simulink subsystem "TransferCaseSSC"  (R2025b)
settings: Solver=VariableStepAuto  StartTime=0.0  StopTime=10.0  RelTol=1e-3
undefined symbols (not defined in the file): PlntTrnsfrCaseCarrDamp, PlntTrnsfrCaseCompStiff, PlntTrnsfrCaseTrqSplitTimeCnst
libraries: sdl_lib x3, nesl_utility_internal x3, fl_lib x2
settings Model: Creator=The MathWorks, Inc.  LastModifiedBy=The MathWorks, Inc.
settings OptimizationCC: ReuseModelBlockBuffer=off
settings RTWCC: GPUComputeCapability=3.5

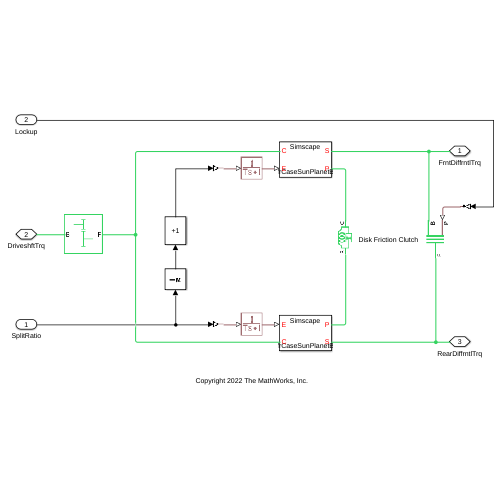
[thumbnail: Simulink's stored preview of the top-level diagram]
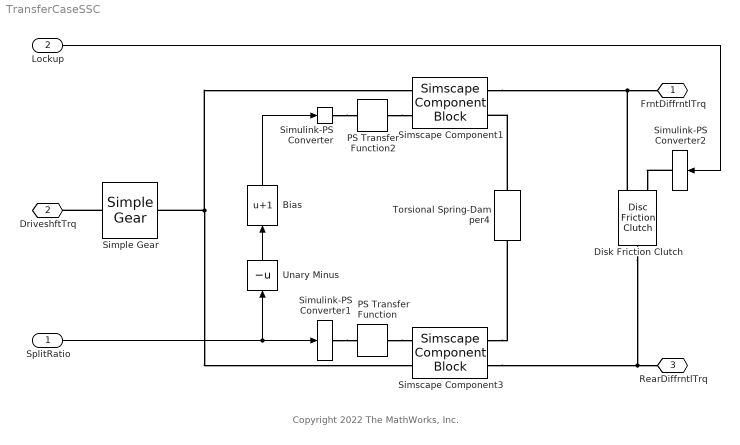
== system TransferCaseSSC ==
  note: Copyright 2022 The MathWorks, Inc.
  SplitRatio : Inport
  Lockup : Inport  Port=2
  Bias : Bias  Bias=1  SaturateOnIntegerOverflow=off
  Disk Friction Clutch : sdl_lib/Clutches/Disc Friction Clutch  geometry_model=sdl.enum.friction_geometry.radius  r_eff=PlntTrnsfrCaseCltchEffRad mm  d_o=150 mm  d_i=100 mm  nS=PlntTrnsfrCaseCltchNumFricSurf  piston_area=PlntTrnsfrCaseCltchEngdPstnArea m^2  unidirectional=sdl.enum.directionality.bidirectional  friction_model=sdl.enum.friction_model_TLU_thermal.fixed  mu_w_vector=[0, 100, 1000] rad/s  temperature_TLU=[280, 300, 320] K  mu_static=PlntTrnsfrCaseCltchStatFric  mu_static_vector=[.4, .38, .36]  mu_coulomb=PlntTrnsfrCaseCltchKinFric  mu_coulomb_vector=[.3, .22, .19]  mu_coulomb_temp_vector=[.3, .28, .25]  mu_coulomb_matrix=[.34, .32, .3; .3, .28, .25; .25, .2, .15]  mu_interp_method=simscape.enum.interpolation.linear  mu_extrap_method=simscape.enum.extrapolation.linear  d_f=PlntTrnsfrCaseCltchDerateFctr  w_tol=PlntTrnsfrCaseCltchVelTol rad/s  pressure_min=PlntTrnsfrCaseCltchEngdThreshPrs Pa  mu_visc=PlntTrnsfrCaseCltchViscDragTrq N*m*s/rad  initial_state_locked=sdl.enum.initial_lock.unlocked  thermal_mass=50 kJ/K  T_init=300 K
      settings: InternalSimscapePortConfiguration="{\"Bottom\":[],\"Left\":[{\"id\":\"P\",\"label\":\"P\",\"type\":\"input\"},{\"id\":\"B\",\"label\":\"B\",\"type\":\"foundation.mechanical.rotational.rotational\"}],\"Right\":[{\"id\":\"F\",\"label\":\"F\",\"type\":\"foundation.mechanical.rotational.rotational\"}],\"Top\":[]}"
  PS Transfer Function : fl_lib/Physical Signals/Linear Operators/PS Transfer Function  transfer_function_type=foundation.enum.transfer_function_type.lag  T=PlntTrnsfrCaseTrqSplitTimeCnst s  T1=2 s  T2=1 s  reset_method=foundation.enum.IntegratorResetSpec.None  initial_condition_spec=foundation.enum.IntegratorICSpec.Internal  y0=PlntTrnsfrCaseTrqSplitRatio
      settings: InternalSimscapePortConfiguration="{\"Bottom\":[],\"Left\":[{\"id\":\"U\",\"label\":\"\",\"type\":\"input\"}],\"Right\":[{\"id\":\"Y\",\"label\":\"\",\"type\":\"output\"}],\"Top\":[]}"
  PS Transfer Function2 : fl_lib/Physical Signals/Linear Operators/PS Transfer Function  transfer_function_type=foundation.enum.transfer_function_type.lag  T=PlntTrnsfrCaseTrqSplitTimeCnst s  T1=2 s  T2=1 s  reset_method=foundation.enum.IntegratorResetSpec.None  initial_condition_spec=foundation.enum.IntegratorICSpec.Internal  y0=PlntTrnsfrCaseTrqSplitRatio
      settings: InternalSimscapePortConfiguration="{\"Bottom\":[],\"Left\":[{\"id\":\"U\",\"label\":\"\",\"type\":\"input\"}],\"Right\":[{\"id\":\"Y\",\"label\":\"\",\"type\":\"output\"}],\"Top\":[]}"
  Simple Gear : sdl_lib/Gears/Simple Gear  ratio=PlntTrnsfrCaseRatio  rotation_direction=sdl.enum.shaftOutputDirection.same  friction_model=sdl.enum.gear_efficiencies_load.constant  T_noload=0.1 N*m  T_nom=5 N*m  efficiency_nom=0.8  efficiency=PlntTrnsfrCaseEff  temperature_TLU=[280, 300, 320] K  load_TLU=[1, 5, 10] N*m  efficiency_TLU=[.95, .9, .85]  efficiency_TLU2=[.85, .8, .75; .95, .9, .85; .85, .8, .7]  w_thr=0.01 rad/s  pwr_thr=PlntTrnsfrCasePwrThresh W  enable_backlash=false  hardstop_model=simscape.enum.hardstop.smooth  backlash_distance=1e-3 mm  r_base=0.1 m  transition=1e-4 mm  backlash_stiffness=1e7 N/m  backlash_damping=1e6 N/(m/s)  coeff_rest=0  v_tol=0.001 m/s  f_tol=0 N  mu_visc=[PlntTrnsfrCaseCarrDamp, PlntTrnsfrCaseCarrDamp] N*m/(rad/s)  thermal_mass=50 J/K  temperature_specify=off  temperature_priority=High  temperature=300 K  temperature_nominal_specify=off  temperature_nominal_value=1  temperature_nominal_unit=K  x_backlash_specify=off  x_backlash_priority=None  x_backlash=0 mm  x_backlash_nominal_specify=off  x_backlash_nominal_value=1  x_backlash_nominal_unit=mm  f_hardstop_specify=off  f_hardstop_priority=None  f_hardstop=0 N  f_hardstop_nominal_specify=off  f_hardstop_nominal_value=1  f_hardstop_nominal_unit=N  v_backlash_specify=off  v_backlash_priority=None  v_backlash=0 m/s  v_backlash_nominal_specify=off  v_backlash_nominal_value=1  v_backlash_nominal_unit=m/s
  Simscape Component1 : SimscapeComponentBlock  SourceFile=TrnsfrCaseSunPlanetBevel  ComponentPath=TrnsfrCaseSunPlanetBevel  ComponentVariants="[\"TrnsfrCaseSunPlanetBevel\"]"  ComponentVariantNames="[\"TrnsfrCaseSunPlanetBevel\"]"  ClassName=TrnsfrCaseSunPlanetBevel  SchemaVersion=1  ratio=PlntTrnsfrCasePlanetSunRatio  assembly_orientation=sdl.enum.sun_planet_bevel_orientation.right  friction_model=sdl.enum.gear_friction.none  efficiency=0.9  temperature_TLU=[280, 300, 320] K  efficiency_TLU=[.95, .9, .85]  pwr_thr=0.001 W  mu_visc=PlntTrnsfrCaseAxl1Damp N*m*s/rad  thermal_mass=50 J/K  temperature_specify=off  temperature_priority=High  temperature=300 K  temperature_nominal_specify=off  temperature_nominal_value=1  temperature_nominal_unit=K
      settings: CopyFcn=simscape.sscblock.internal.componentBlockCallback(gcbh,'COPY')  PreCopyFcn=simscape.sscblock.internal.componentBlockCallback(gcbh,'PRECOPY')  PreDeleteFcn=simscape.sscblock.internal.componentBlockCallback(gcbh,'PREDELETE')  InternalSimscapePortConfiguration="{\"Bottom\":[],\"Left\":[{\"id\":\"ratio2\",\"label\":\"E\",\"type\":\"input\"},{\"id\":\"C\",\"label\":\"C\",\"type\":\"foundation.mechanical.rotational.rotational\"}],\"Right\":[{\"id\":\"P\",\"label\":\"P\",\"type\":\"foundation.mechanical.rotational.rotational\"},{\"id\":\"S\",\"label\":\"S\",\"type\":\"foundation.mechanical.rotational.rotational\"}],\"Top\":[]}"
      mask Type: Sun-Planet Bevel
  Simscape Component3 : SimscapeComponentBlock  SourceFile=TrnsfrCaseSunPlanetBevel  ComponentPath=TrnsfrCaseSunPlanetBevel  ComponentVariants="[\"TrnsfrCaseSunPlanetBevel\"]"  ComponentVariantNames="[\"TrnsfrCaseSunPlanetBevel\"]"  ClassName=TrnsfrCaseSunPlanetBevel  SchemaVersion=1  ratio=PlntTrnsfrCasePlanetSunRatio  assembly_orientation=sdl.enum.sun_planet_bevel_orientation.left  friction_model=sdl.enum.gear_friction.none  efficiency=0.9  temperature_TLU=[280, 300, 320] K  efficiency_TLU=[.95, .9, .85]  pwr_thr=0.001 W  mu_visc=PlntTrnsfrCaseAxl2Damp N*m*s/rad  thermal_mass=50 J/K  temperature_specify=off  temperature_priority=High  temperature=300 K  temperature_nominal_specify=off  temperature_nominal_value=1  temperature_nominal_unit=K
      settings: CopyFcn=simscape.sscblock.internal.componentBlockCallback(gcbh,'COPY')  PreCopyFcn=simscape.sscblock.internal.componentBlockCallback(gcbh,'PRECOPY')  PreDeleteFcn=simscape.sscblock.internal.componentBlockCallback(gcbh,'PREDELETE')  InternalSimscapePortConfiguration="{\"Bottom\":[],\"Left\":[{\"id\":\"ratio2\",\"label\":\"E\",\"type\":\"input\"},{\"id\":\"C\",\"label\":\"C\",\"type\":\"foundation.mechanical.rotational.rotational\"}],\"Right\":[{\"id\":\"P\",\"label\":\"P\",\"type\":\"foundation.mechanical.rotational.rotational\"},{\"id\":\"S\",\"label\":\"S\",\"type\":\"foundation.mechanical.rotational.rotational\"}],\"Top\":[]}"
      mask Type: Sun-Planet Bevel
  Simulink-PS Converter : nesl_utility_internal/Simulink-PS Converter  PhysicalDomain=network_engine_domain  SubClassName=ps_input  LeftPortType=input  RightPortType=output  PseudoPeriodic=off  Frequencies=[]  NoiseDistribution=none  NoiseParameters=[]  Unit=1  AffineConversion=off  FilteringAndDerivatives=zero  SimscapeFilterOrder=1  InputFilterTimeConstant=0.001  UdotUserProvided=0
  Simulink-PS Converter1 : nesl_utility_internal/Simulink-PS Converter  PhysicalDomain=network_engine_domain  SubClassName=ps_input  LeftPortType=input  RightPortType=output  PseudoPeriodic=off  Frequencies=[]  NoiseDistribution=none  NoiseParameters=[]  Unit=1  AffineConversion=off  FilteringAndDerivatives=zero  SimscapeFilterOrder=1  InputFilterTimeConstant=0.001  UdotUserProvided=1
  Simulink-PS Converter2 : nesl_utility_internal/Simulink-PS Converter  PhysicalDomain=network_engine_domain  SubClassName=ps_input  LeftPortType=input  RightPortType=output  PseudoPeriodic=off  Frequencies=[]  NoiseDistribution=none  NoiseParameters=[]  Unit=Pa  AffineConversion=off  FilteringAndDerivatives=filter  SimscapeFilterOrder=1  InputFilterTimeConstant=0.001  UdotUserProvided=0
  Torsional Spring-Damper4 : sdl_lib/Couplings & Drives/Torsional Spring-Damper  k=PlntTrnsfrCaseCompStiff N*m/rad  mu_visc=PlntTrnsfrCaseCompViscFric N*m/(rad/s)  trq_coulomb=PlntTrnsfrCaseCompCoulFricTrq N*m  static_kinetic_ratio=PlntTrnsfrCaseCompStatKinFricRatio  w_tol=PlntTrnsfrCaseCompVelTol rad/s  model_hardstop=sdl.enum.hardStopOffOn.off  upper_bound=10 deg  lower_bound=-10 deg  hardstop_model=simscape.enum.hardstop.smooth  k_endstop=1e6 N*m/rad  D_endstop=10 N*m/(rad/s)  transition=0.001 rad  coeff_rest=0.7  w_tol_hardstop=0.1 rad/s  trq_tol=0.001 N*m  x0=PlntTrnsfrCaseCompInitDef rad
      settings: InternalSimscapePortConfiguration="{\"Bottom\":[],\"Left\":[{\"id\":\"R\",\"label\":\"R\",\"type\":\"foundation.mechanical.rotational.rotational\"}],\"Right\":[{\"id\":\"C\",\"label\":\"C\",\"type\":\"foundation.mechanical.rotational.rotational\"}],\"Top\":[]}"
  Unary Minus : UnaryMinus
  FrntDiffrntlTrq : PMIOPort  Side=Left
  DriveshftTrq : PMIOPort  Port=2  Side=Left
  RearDiffrntlTrq : PMIOPort  Port=3  Side=Left
  wires:
  SplitRatio/1 -> Simulink-PS Converter1/1, Unary Minus/1
  Bias/1 -> Simulink-PS Converter/1
  Unary Minus/1 -> Bias/1
  Lockup/1 -> Simulink-PS Converter2/1
  connections:
  Simscape Component3/RConn2 -- RearDiffrntlTrq/RConn1 -- Disk Friction Clutch/RConn1
  Simscape Component1/RConn2 -- FrntDiffrntlTrq/RConn1 -- Disk Friction Clutch/LConn2
  Simple Gear/RConn1 -- Simscape Component1/LConn2 -- Simscape Component3/LConn2
  PS Transfer Function2/RConn1 -- Simscape Component1/LConn1
  Simple Gear/LConn1 -- DriveshftTrq/RConn1
  Simscape Component3/RConn1 -- Torsional Spring-Damper4/LConn1
  Simulink-PS Converter2/RConn1 -- Disk Friction Clutch/LConn1
  Simulink-PS Converter1/RConn1 -- PS Transfer Function/LConn1
  Simulink-PS Converter/RConn1 -- PS Transfer Function2/LConn1
  Torsional Spring-Damper4/RConn1 -- Simscape Component1/RConn1
  PS Transfer Function/RConn1 -- Simscape Component3/LConn1
